simulink model "sysgenCORDICSinCos"  (Simulink 7.7)
settings: Solver=ode45  StartTime=0.0  StopTime=500  RelTol=1e-3
values from neighbouring files (symbols this model uses):
  blue = blue(1:(min_x*min_y))    [makematrix.m]    (also in rgb.mat = [0 0 0 255 255 255 255 255 255 0 0 0 ... (256 elements, 256x)
undefined symbols (not defined in the file or in its folder): Error_Measurement, sysgenCORDIC_lib
libraries: xbsIndex_r4 x95, dspobslib x9, dspstat3 x4, dspswit3 x2, xbsCopyrightNotice_r4 x1, simulink x1
(part 1 of 2)
settings Model: Creator=alexc  LastModifiedBy=douangp
settings DataIOCC: SignalLoggingName=sigsOut
settings OptimizationCC: BlockReduction=off  BooleanDataType=off  InlineInvariantSignals=on  InitFltsAndDblsToZero=on
settings DebuggingCC: SaveWithParameterizedLinksMsg=none  SignalResolutionControl=TryResolveAllWithWarning  SolverPrmCheckMsg=none  MultiTaskDSMMsg=warning  MultiTaskCondExecSysMsg=none  StrictBusMsg=None
settings HardwareCC: TargetUnknown=on
settings RTWCC: IncludeERTFirstTime=on
settings GRTTargetCC: TargetFcnLib=ansi_tfl_tmw.mat

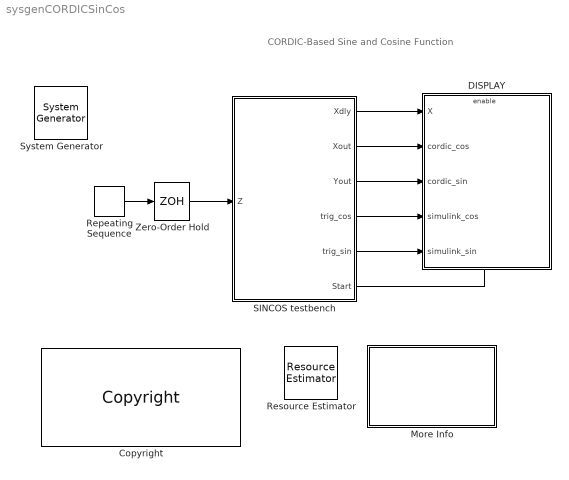
== system sysgenCORDICSinCos ==
  note: CORDIC-Based Sine and Cosine Function
  " System Generator" : xbsIndex_r4/ System Generator  Tag=genX  SystemSampleTime=-1  xilinxfamily=kintex7  part=xc7k325t  speed=-1  package=ffg900  synthesis_tool=XST  clock_wrapper=Clock Enables  directory=./netlist_sysgenCordicSinCos  proj_type=Project Navigator  Synth_file=XST Defaults  Impl_file=ISE Defaults  testbench=off  simulink_period=1  sysclk_period=5  dcm_input_clock_period=100  incr_netlist=off  trim_vbits=Everywhere in SubSystem  dbl_ovrd=According to Block Masks  core_generation=Not Needed - Already Generated  run_coregen=off  deprecated_control=off  eval_field=0  block_type=sysgen
      settings: block_version=9.2.00
  Copyright : xbsCopyrightNotice_r4/Copyright  copyrighttext="Copyright (c) 2011  by  Xilinx, Inc. All rights reserved.<br><br>This file contains proprietary, confidential information of Xilinx, Inc., is distributed under license from Xilinx, Inc., and may be used, copied and/or disclosed only pursuant to the terms of a valid license agreement with Xilinx, Inc. Xilinx hereby grants you a license to use this file solely for design, simulation, implementation and creation of design files limited to Xilinx devices or technologies. Use with non-Xilinx devices or technologies is expressly prohibited and immediately terminates your license unless covered by a separate agreement.<br><br>Xilinx is providing this design, code, or information \"as-is\" solely for use in developing programs and solutions for Xilinx devices, with no obligation on the part of Xilinx to provide support. By providing this design, code, or information as one possible implementation of this feature, application or standard, Xilinx is making no representation that this implementation is free from any claims of infringement. You are responsible for obtaining any rights you may require for your implementation. Xilinx expressly disclaims any warranty whatsoever with respect to the adequacy of the implementation, including but not limited to any warranties or representations that this implementation is free from claims of infringement, implied warranties of merchantability or fitness for a particular purpose.<br><br>Xilinx products are not intended for use in life support appliances, devices, or systems. Use in such applications is expressly prohibited.<br><br>Any modifications that are made to the Source Code are done at the user's sole risk and will be unsupported.<br><br>This copyright and support notice must be retained as part of this text at all times. (c) Copyright 1995-2011 Xilinx, Inc. All rights reserved."  block_type=copyright
      settings: block_version=10.1.00
      settings: infoedit=|
      | Copyright(C) 2008 by  Xilinx, Inc. All rights reserved.<br>
      | <br>
      | This file contains proprietary, confidential information of Xilinx, Inc., is distributed under license
      | from Xilinx, Inc., and may be used, copied and/or disclosed only pursuant to the terms of a valid license
      | agreement with Xilinx, Inc. Xilinx hereby grants you a license to use this file solely for design,
      | simulation, implementation and creation of design files limited to Xilinx devices or technologies. Use
      | with non-Xilinx devices or technologies is expressly prohibited and immediately terminates your license
      | unless covered by a separate agreement.<br>
      | <br>
      | Xilinx is providing this design, code, or information "as-is" solely for use in developing programs and
      | solutions for Xilinx devices, with no obligation on the part of Xilinx to provide support. By providing
      | this design, code, or information as one possible implementation of this feature, application or standard,
      | Xilinx is making no representation that this implementation is free from any claims of infringement. You
      | are responsible for obtaining any rights you may require for your implementation. Xilinx expressly disclaims
      | any warranty whatsoever with respect to the adequacy of the implementation, including but not limited to any
      | warranties or representations that this implementation is free from claims of infringement, implied warranties
      | of merchantability or fitness for a particular purpose.<br>
      | <br>
      | Xilinx products are not intended for use in life support appliances, devices, or systems. Use in such
      | applications is expressly prohibited.<br>
      | <br>
      | Any modifications that are made to the Source Code are done at the user's sole risk and will be unsupported.<br>
      | <br>
      | This copyright and support notice must be retained as part of this text at all times.
      | (c) Copyright 1995-2008 Xilinx, Inc. All rights reserved.
  DISPLAY : Subsystem  TreatAsAtomicUnit=on
  More Info : Subsystem
      mask Display: disp('Double click\n for\n more information.')
  Repeating Sequence : simulink/Sources/Repeating Sequence  SystemSampleTime=-1  rep_seq_t=0:1:201  rep_seq_y=-pi:1/32:pi
  Resource Estimator : xbsIndex_r4/Resource Estimator  Tag=resEstTag  Slices=324  FFs=532  BRAMs=0  LUTs=556  IOBs=48  EBMs=0  TBUFs=0  xl_use_estimator_area=off  est_options=Estimate  xl_estimator_area=[324 532 0 556 48 0 0]  mrp_directory=./sysgenCORDIC_work_test  simulink_period=1  block_type=resource_estimator
      settings: AttributesFormatString=Resource\nEstimator  block_version=9.2.00
  SINCOS testbench : Subsystem  mask{pe_stages=8, pe_nbits=16, pe_binpt=13}
      mask prompts: pe_stages "Number of Processing Stages"; pe_nbits "Number of X, Y, Z Bits"; pe_binpt "X, Y, Z Binary Point Position"
      mask help: CORDIC processor and Simulink conformance testbench. Block parameters allow customization of the CORDIC processor. The number of iteration stages (and resultant output accuracy) and the processor arithmetic precision are controlled by the mask customization.
      mask init:
      | [bg,fg] = xlcmap('XBlock',0);
      | iPos = get_param(gcb,'Position');
      | iWidth=iPos(3)-iPos(1); iHeight=iPos(4)-iPos(2);
      | iCx=iWidth/2;
      | iCy=iHeight/2;
      | [logoX, logoY] = xlogo(iPos);
      | 
      | latency = pe_stages + 5;
      | str = sprintf('-%d',latency);
      mask Help:
      | This design implements a fully parallel CORDIC  (COordinate Rotation DIgital Computer) algorithm in rotational mode that computes
      | the sine and cosine of the input angle z between +/- pi.
      | </p>
      | The CORDIC algorithm is attractive for an FPGA implementation because it consists primarily of shift and add operations.
      | An N-bit adder/subtractor  requiries only N/2 logic slices.  The CORDIC subsystem is masked, and allows customization of bit precision,
      | the number of processing elements (PEs) in the CORDIC engine and the ability to pieline each individual stage.  With eight PEs, the design occupies 503 LUTs (49%),
      | 412 flip-flops (40%), and 272 slices (53%) of a Xilinx xc2v80-5 part. The maximum clock frequency is approximately 230.04 MHz (Device speed data version:
      | PRODUCTION 1.121 2005-11-04, ISE 8.1i software, VHDL synthesized with XST).
      | </p>
      | The CORDIC subsystem is suitable for reuse as a standalone component.
      | </p>
      | <ul>
      | References:
      | <li>J. E. Volder, "The CORDIC Trigonometric Computing Technique", IRE Trans. On Electronic Computers, Vol. EC-8,  1959, pp. 330-334.</li>
      | <li>J. S. Walther, "A Unified Algorithm for Elementary Functions", Spring Joint Computer Conference (1971) pp. 379-385.</li>
      | <li>Yu Hen Hu, "CORDIC-Based VLSI Architectures for Digital Signal Processing", IEEE Signal Processing Magazine, pp. 17-34, July 1992.</li>
      | </ul>
      mask Display:
      | patch([0 iWidth iWidth 0],[0 0 iHeight iHeight] , bg);
      | patch(logoX,logoY , fg);
      | text(iCx-6,iCy,'z');
      | text(iCx,iCy+4,str);
      | port_label('input',1,'z');
      | port_label('output',1,'z_dly');
      | port_label('output',2,'cordic_cos');
      | port_label('output',3,'cordic_sine');
      | port_label('output',4,'simulink_cos');
      | port_label('output',5,'simulink_sin');
      | port_label('output',6,'Start');
      | plot([0 0 iWidth iWidth 0], [0 iHeight iHeight 0 0]);
  Zero-Order Hold : ZeroOrderHold
  wires:
  SINCOS testbench/1(Xdly) -> DISPLAY/1(X)
  SINCOS testbench/4(trig_cos) -> DISPLAY/4(simulink_cos)
  SINCOS testbench/5(trig_sin) -> DISPLAY/5(simulink_sin)
  SINCOS testbench/6(Start) -> DISPLAY/Enable
  Zero-Order Hold/1 -> SINCOS testbench/1(Z)
  Repeating Sequence/1 -> Zero-Order Hold/1
  SINCOS testbench/2(Xout) -> DISPLAY/2(cordic_cos)
  SINCOS testbench/3(Yout) -> DISPLAY/3(cordic_sin)

== system sysgenCORDICSinCos/DISPLAY ==
  note: This subsystem compares the fixed-point CORDIC output with double-precision functions computed in Simulink. The CORDIC OVERLAY scope
      | displays the original input signals and the superposition of the respective output signals.  The Error Measurement subsystems provide additional
      | comparative information.  This enabled subsystem is activated after the number of sample periods equal to the latency of the CORDIC processor.
  X : Inport
  cordic_cos : Inport  Port=2
  cordic_sin : Inport  Port=3
  simulink_cos : Inport  Port=4
  simulink_sin : Inport  Port=5
  Enable : EnablePort
  CORDIC  OVERLAY : Scope  NumInputPorts=3
      settings: TimeRange=500  YMin=-4~-1~-1.5  YMax=4~1.5~1.5
  Mux : Mux  Inputs=2
  Mux1 : Mux  Inputs=2
  cos  Error Measurement : Subsystem  AncestorBlock=sysgenCORDIC_lib/Error_Measurement
      mask Type: Error Measurement
  sin  Error Measurement : Subsystem
      mask Type: Error Measurement
  wires:
  cordic_cos/1 -> Mux/1, cos  Error Measurement/1(In1)
  simulink_cos/1 -> Mux/2, cos  Error Measurement/2(In2)
  X/1 -> CORDIC  OVERLAY/1
  cordic_sin/1 -> Mux1/1, sin  Error Measurement/1(In1)
  simulink_sin/1 -> Mux1/2, sin  Error Measurement/2(In2)
  Mux1/1 -> CORDIC  OVERLAY/3
  Mux/1 -> CORDIC  OVERLAY/2

== system sysgenCORDICSinCos/More Info ==
  note: This design implements a fully parallel CORDIC  (COordinate Rotation DIgital Computer) algorithm in rotational mode that computes
      | the sine and cosine of the input angle z between +/- pi.
      |
      | The CORDIC algorithm is attractive for an FPGA implementation because it consists primarily of shift and add operations.
      | An N-bit adder/subtractor  requiries only N/2 logic slices.  The CORDIC subsystem is masked, and allows customization of bit precision,
      | the number of processing elements (PEs) in the CORDIC engine and the ability to pieline each individual stage.
      |
      | References:
      | J. E. Volder, "The CORDIC Trigonometric Computing Technique", IRE Trans. On Electronic Computers, Vol. EC-8,  1959, pp. 330-334.
      | J. S. Walther, "A Unified Algorithm for Elementary Functions", Spring Joint Computer Conference (1971) pp. 379-385.
      | Yu Hen Hu, "CORDIC-Based VLSI Architectures for Digital Signal Processing", IEEE Signal Processing Magazine, pp. 17-34, July 1992.
  note: CORDIC-Based Sine and Cosine Function

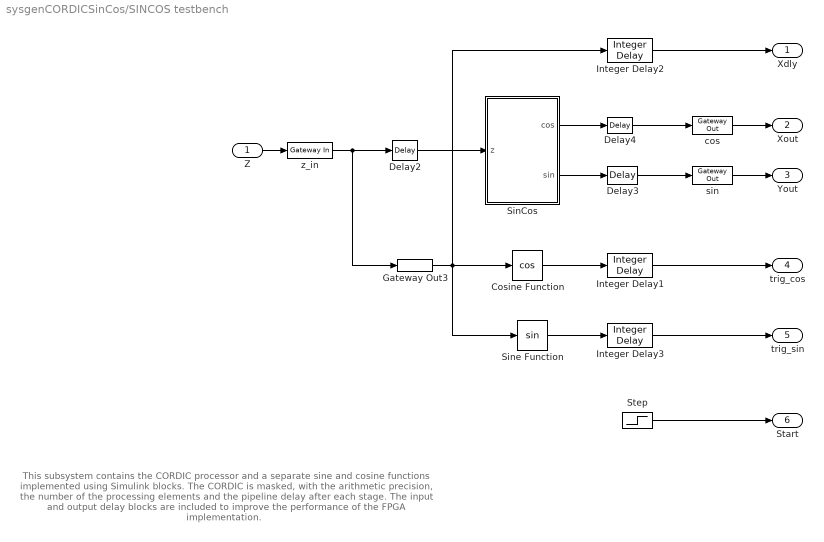
== system sysgenCORDICSinCos/SINCOS testbench ==
  note: This subsystem contains the CORDIC processor and a separate sine and cosine functions implemented using Simulink blocks.
      | The CORDIC is masked, with the arithmetic precision, the number of the processing elements and the pipeline delay after each
      | stage. The input and output delay blocks are included to improve the performance of the FPGA implementation.
  Z : Inport
  Cosine Function : Trigonometry  Operator=cos
  Delay2 : xbsIndex_r4/Delay  rst=off  infoeditControl=Selection of Reset will increase slice count due to use of real FFs and instead of SRLs  en=off  latency=1  dbl_ovrd=off  reg_retiming=off  block_type=delay
      settings: infoedit="Delay line having  configurable length.<P><P>Hardware notes: A delay line is a chain, each link of which is an SRL16 followed by a flip-flop. If register retiming is enabled, the delay line is a chain of flip-flops."  xl_area=[8 16 0 0 0 0 0]  block_version=VER_STRING_GOES_HERE
  Delay3 : xbsIndex_r4/Delay  rst=off  infoeditControl=Selection of Reset will increase slice count due to use of real FFs and instead of SRLs  en=off  latency=1  dbl_ovrd=off  reg_retiming=off  block_type=delay
      settings: infoedit="Delay line having  configurable length.<P><P>Hardware notes: A delay line is a chain, each link of which is an SRL16 followed by a flip-flop. If register retiming is enabled, the delay line is a chain of flip-flops."  xl_area=[8 16 0 0 0 0 0]  block_version=VER_STRING_GOES_HERE
  Delay4 : xbsIndex_r4/Delay  rst=off  infoeditControl=Selection of Reset will increase slice count due to use of real FFs and instead of SRLs  en=off  latency=1  dbl_ovrd=off  reg_retiming=off  block_type=delay
      settings: infoedit="Delay line having  configurable length.<P><P>Hardware notes: A delay line is a chain, each link of which is an SRL16 followed by a flip-flop. If register retiming is enabled, the delay line is a chain of flip-flops."  xl_area=[8 16 0 0 0 0 0]  block_version=VER_STRING_GOES_HERE
  Gateway Out3 : xbsIndex_r4/Gateway Out  hdl_port=off  timing_constraint=None  locs_specified=off  LOCs={}  block_type=gatewayout
      settings: infoedit="Gateway out block.  Converts Xilinx fixed point inputs into ouputs of type Simulink integer, double, or fixed point.<P><P>Hardware notes:  In hardware these blocks become top level output ports or are discarded, depending on how they are configured."  xl_area=[0 0 0 0 0 0 0]  block_version=VER_STRING_GOES_HERE
  Integer Delay1 : dspobslib/Integer Delay  delay=latency  ic=0  reset_popup=None
  Integer Delay2 : dspobslib/Integer Delay  delay=latency  ic=0  reset_popup=None
  Integer Delay3 : dspobslib/Integer Delay  delay=latency  ic=0  reset_popup=None
  SinCos : Subsystem  mask{pe_stages=pe_stages, pe_nbits=pe_nbits, pe_binpt=pe_binpt, sg_icon_stat=80,126,1,3,white,blue,0,,right}
      mask prompts: pe_stages "Stages"; pe_nbits "Number of bits"; pe_binpt "Binary point position"; sg_icon_stat "Mask Parameter 4:"
      mask init:
      | xBlock(struct('source', str2func('cordic_sincos_script'), 'toplevel', gcb, 'depend', {{'cordic_sincos_script'}}), {pe_stages, pe_nbits, pe_binpt});
      mask Display:
      | fprintf('','COMMENT: begin icon graphics');
      | patch([0 70 70 0 ],[0 0 104 104 ],[0.77 0.82 0.91]);
      | patch([17 5 21 5 17 35 40 45 65 49 34 23 39 23 34 49 65 45 40 35 17 ],[25 37 53 69 81 81 76 81 81 65 80 69 53 37 26 41 25 25 30 25 25 ],[0.98 0.96 0.92]);
      | plot([0 70 70 0 0 ],[0 0 104 104 0 ]);
      | fprintf('','COMMENT: end icon graphics');
      | fprintf('','COMMENT: begin icon text');
      | color('black');port_label('input',1,'z');
      | color('black');port_label('output',1,'cos');
      | color('black');port_label('output',2,'sin');
      | fprintf('','COMMENT: end icon text');
  Sine Function : Trigonometry
  Step : Step  Time=latency  SampleTime=1
  cos : xbsIndex_r4/Gateway Out  hdl_port=on  timing_constraint=None  locs_specified=off  LOCs={}  block_type=gatewayout
      settings: infoedit="Gateway out block.  Converts Xilinx fixed point inputs into ouputs of type Simulink integer, double, or fixed point.<P><P>Hardware notes:  In hardware these blocks become top level output ports or are discarded, depending on how they are configured."  xl_area=[0 0 0 0 16 0 0]  block_version=VER_STRING_GOES_HERE
  sin : xbsIndex_r4/Gateway Out  hdl_port=on  timing_constraint=None  locs_specified=off  LOCs={}  block_type=gatewayout
      settings: infoedit="Gateway out block.  Converts Xilinx fixed point inputs into ouputs of type Simulink integer, double, or fixed point.<P><P>Hardware notes:  In hardware these blocks become top level output ports or are discarded, depending on how they are configured."  xl_area=[0 0 0 0 16 0 0]  block_version=VER_STRING_GOES_HERE
  z_in : xbsIndex_r4/Gateway In  gui_display_data_type=Fixed-point  arith_type="Signed  (2's comp)"  n_bits=pe_nbits  bin_pt=pe_binpt  preci_type=Single  exp_width=8  frac_width=24  quantization="Round  (unbiased: +/- Inf)"  overflow=Saturate  period=1  dbl_ovrd=off  timing_constraint=None  locs_specified=off  LOCs={}  hdl_port=on  block_type=gatewayin
      settings: infoedit="Gateway in block.  Converts inputs of type Simulink integer, double and fixed point to  Xilinx fixed point type.<P><P>Hardware notes:  In hardware these blocks become top level input ports."  xl_area=[0 0 0 0 16 0 0]  block_version=VER_STRING_GOES_HERE
  Xdly : Outport
  Xout : Outport  Port=2
  Yout : Outport  Port=3
  trig_cos : Outport  Port=4
  trig_sin : Outport  Port=5
  Start : Outport  Port=6
  wires:
  Gateway Out3/1 -> Sine Function/1, Cosine Function/1, Integer Delay2/1
  Step/1 -> Start/1
  Integer Delay3/1 -> trig_sin/1
  Integer Delay1/1 -> trig_cos/1
  sin/1 -> Yout/1
  cos/1 -> Xout/1
  Sine Function/1 -> Integer Delay3/1
  Delay4/1 -> cos/1
  Z/1 -> z_in/1
  Integer Delay2/1 -> Xdly/1
  Delay3/1 -> sin/1
  Delay2/1 -> SinCos/1(z)
  Cosine Function/1 -> Integer Delay1/1
  z_in/1 -> Gateway Out3/1, Delay2/1
  SinCos/1(cos) -> Delay4/1
  SinCos/2(sin) -> Delay3/1

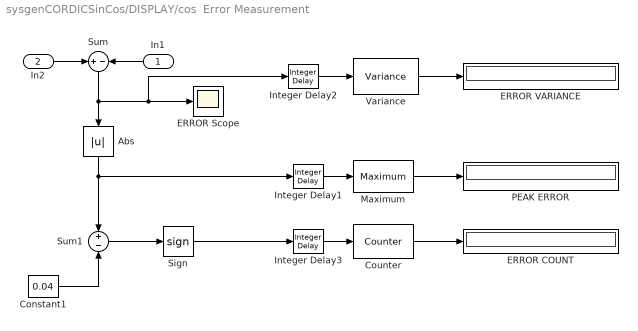
== system sysgenCORDICSinCos/DISPLAY/cos  Error Measurement ==
  In1 : Inport
  In2 : Inport  Port=2
  Abs : Abs  SaturateOnIntegerOverflow=on
  Constant1 : Constant  Value=0.04
  Counter : dspswit3/Counter  Direction=Up  CountEvent=Rising edge  CounterSize=User defined  MaxCount=200000000  InitialCount=0  Output=Count  HitValue=32  ResetInput=off  SamplesPerFrame=1  Ts=1  CntDtype=double  HitDtype=Logical
  ERROR Scope : Scope
      settings: TimeRange=10000  YMin=-0.0006  YMax=0.0005  SaveName=ScopeData2
  ERROR COUNT : Display
      settings: Format=long_e
  ERROR VARIANCE : Display
      settings: Format=long_e
  Integer Delay1 : dspobslib/Integer Delay  delay=1  ic=0  reset_popup=None
  Integer Delay2 : dspobslib/Integer Delay  delay=1  ic=0  reset_popup=None
  Integer Delay3 : dspobslib/Integer Delay  delay=1  ic=0  reset_popup=None
  Maximum : dspstat3/Maximum  fcn=Running  reset=None  InputProcessing=Inherited (this choice will be removed - see release notes)  indexBase=One  operateOver=Each column  Dimension=1  colComp=on  operation=maximum  roiEnable=off  roiType=Rectangles  roiPortion=Entire ROI  roiOutput=Individual statistics for each ROI  roiFlag=off  accumDataTypeStr=Inherit: Same as product output  accumLastDataTypeStr=Inherit: Same as product output  roundingMode=Floor  overflowMode=off
  PEAK ERROR : Display
      settings: Format=long_e
  Sign : Signum
  Sum : Sum  Inputs=+-  SaturateOnIntegerOverflow=on  InputSameDT=on  OutDataTypeStr=Inherit: Same as first input
  Sum1 : Sum  Inputs=+-  SaturateOnIntegerOverflow=on  InputSameDT=on  OutDataTypeStr=Inherit: Same as first input
  Variance : dspstat3/Variance  run=on  reset_popup=None  InputProcessing=Inherited (this choice will be removed - see release notes)  directionMode=Each column  dimension=1  treatSBRowAsCol=on  roiEnable=off  roiType=Rectangles  roiPortion=Entire ROI  roiOutput=Individual statistics for each ROI  roiFlag=off  roundingMode=Floor  overflowMode=off
  wires:
  Sum/1 -> Abs/1, ERROR Scope/1, Integer Delay2/1
  Constant1/1 -> Sum1/2
  Abs/1 -> Sum1/1, Integer Delay1/1
  Sum1/1 -> Sign/1
  Sign/1 -> Integer Delay3/1
  Counter/1 -> ERROR COUNT/1
  Variance/1 -> ERROR VARIANCE/1
  Maximum/1 -> PEAK ERROR/1
  Integer Delay3/1 -> Counter/1
  Integer Delay1/1 -> Maximum/1
  Integer Delay2/1 -> Variance/1
  In1/1 -> Sum/2
  In2/1 -> Sum/1

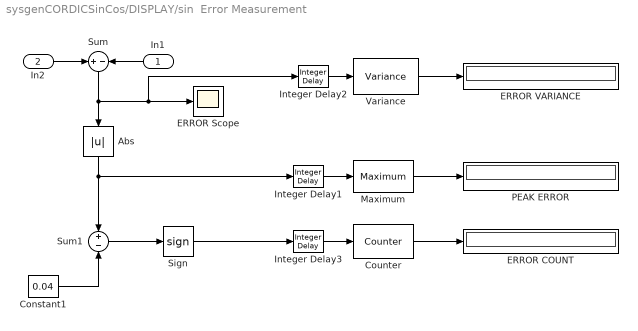
== system sysgenCORDICSinCos/DISPLAY/sin  Error Measurement ==
  In1 : Inport
  In2 : Inport  Port=2
  Abs : Abs  SaturateOnIntegerOverflow=on
  Constant1 : Constant  Value=0.04
  Counter : dspswit3/Counter  Direction=Up  CountEvent=Rising edge  CounterSize=User defined  MaxCount=200000000  InitialCount=0  Output=Count  HitValue=32  ResetInput=off  SamplesPerFrame=1  Ts=1  CntDtype=double  HitDtype=Logical
  ERROR Scope : Scope
      settings: TimeRange=10000  YMin=-0.0006  YMax=0.0005  SaveName=ScopeData2
  ERROR COUNT : Display
      settings: Format=long_e
  ERROR VARIANCE : Display
      settings: Format=long_e
  Integer Delay1 : dspobslib/Integer Delay  delay=1  ic=0  reset_popup=None
  Integer Delay2 : dspobslib/Integer Delay  delay=1  ic=0  reset_popup=None
  Integer Delay3 : dspobslib/Integer Delay  delay=1  ic=0  reset_popup=None
  Maximum : dspstat3/Maximum  fcn=Running  reset=None  InputProcessing=Inherited (this choice will be removed - see release notes)  indexBase=One  operateOver=Each column  Dimension=1  colComp=on  operation=maximum  roiEnable=off  roiType=Rectangles  roiPortion=Entire ROI  roiOutput=Individual statistics for each ROI  roiFlag=off  accumDataTypeStr=Inherit: Same as product output  accumLastDataTypeStr=Inherit: Same as product output  roundingMode=Floor  overflowMode=off
  PEAK ERROR : Display
      settings: Format=long_e
  Sign : Signum
  Sum : Sum  Inputs=+-  SaturateOnIntegerOverflow=on  InputSameDT=on  OutDataTypeStr=Inherit: Same as first input
  Sum1 : Sum  Inputs=+-  SaturateOnIntegerOverflow=on  InputSameDT=on  OutDataTypeStr=Inherit: Same as first input
  Variance : dspstat3/Variance  run=on  reset_popup=None  InputProcessing=Inherited (this choice will be removed - see release notes)  directionMode=Each column  dimension=1  treatSBRowAsCol=on  roiEnable=off  roiType=Rectangles  roiPortion=Entire ROI  roiOutput=Individual statistics for each ROI  roiFlag=off  roundingMode=Floor  overflowMode=off
  wires:
  Sum/1 -> Abs/1, ERROR Scope/1, Integer Delay2/1
  Constant1/1 -> Sum1/2
  Abs/1 -> Sum1/1, Integer Delay1/1
  Sum1/1 -> Sign/1
  Sign/1 -> Integer Delay3/1
  Counter/1 -> ERROR COUNT/1
  Variance/1 -> ERROR VARIANCE/1
  Maximum/1 -> PEAK ERROR/1
  Integer Delay3/1 -> Counter/1
  Integer Delay1/1 -> Maximum/1
  Integer Delay2/1 -> Variance/1
  In1/1 -> Sum/2
  In2/1 -> Sum/1

== system sysgenCORDICSinCos/SINCOS testbench/SinCos ==
  z : Inport
  Constant2 : xbsIndex_r4/Constant  const=0.607253030192621  gui_display_data_type=Fixed-point  arith_type=Signed (2's comp)  n_bits=16  bin_pt=13  preci_type=Single  exp_width=8  frac_width=24  explicit_period=off  period=1  equ=P=C  opselect=C  inp2=PCIN>>17  opr=+  inp1=P  carry=CIN  dbl_ovrd=off  block_type=constant
  Constant3 : xbsIndex_r4/Constant  const=0  gui_display_data_type=Fixed-point  arith_type=Signed (2's comp)  n_bits=16  bin_pt=13  preci_type=Single  exp_width=8  frac_width=24  explicit_period=off  period=1  equ=P=C  opselect=C  inp2=PCIN>>17  opr=+  inp1=P  carry=CIN  dbl_ovrd=off  block_type=constant
  Delay1 : xbsIndex_r4/Delay  rst=off  infoeditControl=Selection of Reset will increase slice count due to use of real FFs and instead of SRLs  en=off  latency=9  dbl_ovrd=off  reg_retiming=off  block_type=delay
  Delay2 : xbsIndex_r4/Delay  rst=off  infoeditControl=Selection of Reset will increase slice count due to use of real FFs and instead of SRLs  en=off  latency=10  dbl_ovrd=off  reg_retiming=off  block_type=delay
  fine_angle_pe : Subsystem
  quandrant_correct : Subsystem
  quandrant_map : Subsystem
  cos : Outport
  sin : Outport  Port=2
  wires:
  quandrant_correct/2(sine) -> sin/1
  quandrant_correct/1(cosine) -> cos/1
  Delay2/1 -> quandrant_correct/4(sgn_z)
  Delay1/1 -> quandrant_correct/3(angle_map)
  fine_angle_pe/2(out1) -> quandrant_correct/2(s)
  fine_angle_pe/1(out0) -> quandrant_correct/1(c)
  quandrant_map/3(sgn_z) -> Delay2/1
  quandrant_map/2(angle_map) -> Delay1/1
  quandrant_map/1(zo) -> fine_angle_pe/3(in2)
  Constant3/1 -> fine_angle_pe/2(in1)
  Constant2/1 -> fine_angle_pe/1(in0)
  z/1 -> quandrant_map/1(z)

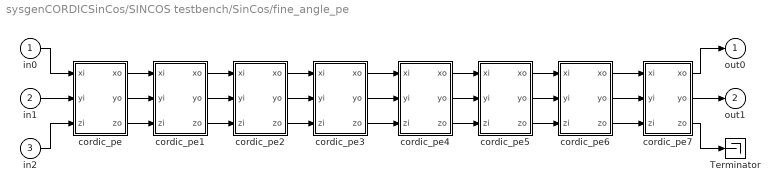
== system sysgenCORDICSinCos/SINCOS testbench/SinCos/fine_angle_pe ==
  in0 : Inport
  in1 : Inport  Port=2
  in2 : Inport  Port=3
  Terminator : Terminator
  cordic_pe : Subsystem
  cordic_pe1 : Subsystem
  cordic_pe2 : Subsystem
  cordic_pe3 : Subsystem
  cordic_pe4 : Subsystem
  cordic_pe5 : Subsystem
  cordic_pe6 : Subsystem
  cordic_pe7 : Subsystem
  out0 : Outport
  out1 : Outport  Port=2
  wires:
  cordic_pe7/3(zo) -> Terminator/1
  cordic_pe7/2(yo) -> out1/1
  cordic_pe7/1(xo) -> out0/1
  cordic_pe6/3(zo) -> cordic_pe7/3(zi)
  cordic_pe6/2(yo) -> cordic_pe7/2(yi)
  cordic_pe6/1(xo) -> cordic_pe7/1(xi)
  cordic_pe5/3(zo) -> cordic_pe6/3(zi)
  cordic_pe5/2(yo) -> cordic_pe6/2(yi)
  cordic_pe5/1(xo) -> cordic_pe6/1(xi)
  cordic_pe4/3(zo) -> cordic_pe5/3(zi)
  cordic_pe4/2(yo) -> cordic_pe5/2(yi)
  cordic_pe4/1(xo) -> cordic_pe5/1(xi)
  cordic_pe3/3(zo) -> cordic_pe4/3(zi)
  cordic_pe3/2(yo) -> cordic_pe4/2(yi)
  cordic_pe3/1(xo) -> cordic_pe4/1(xi)
  cordic_pe2/3(zo) -> cordic_pe3/3(zi)
  cordic_pe2/2(yo) -> cordic_pe3/2(yi)
  cordic_pe2/1(xo) -> cordic_pe3/1(xi)
  cordic_pe1/3(zo) -> cordic_pe2/3(zi)
  cordic_pe1/2(yo) -> cordic_pe2/2(yi)
  cordic_pe1/1(xo) -> cordic_pe2/1(xi)
  cordic_pe/3(zo) -> cordic_pe1/3(zi)
  cordic_pe/2(yo) -> cordic_pe1/2(yi)
  cordic_pe/1(xo) -> cordic_pe1/1(xi)
  in2/1 -> cordic_pe/3(zi)
  in1/1 -> cordic_pe/2(yi)
  in0/1 -> cordic_pe/1(xi)

== system sysgenCORDICSinCos/SINCOS testbench/SinCos/quandrant_correct ==
  c : Inport
  s : Inport  Port=2
  angle_map : Inport  Port=3
  sgn_z : Inport  Port=4
  Mux1 : xbsIndex_r4/Mux  inputs=2  en=off  latency=0  precision=Full  arith_type=Unsigned  n_bits=16  bin_pt=14  quantization=Truncate  overflow=Wrap  dbl_ovrd=off  block_type=mux
  Mux2 : xbsIndex_r4/Mux  inputs=2  en=off  latency=0  precision=Full  arith_type=Unsigned  n_bits=16  bin_pt=14  quantization=Truncate  overflow=Wrap  dbl_ovrd=off  block_type=mux
  Mux3 : xbsIndex_r4/Mux  inputs=2  en=off  latency=1  precision=Full  arith_type=Unsigned  n_bits=16  bin_pt=14  quantization=Truncate  overflow=Wrap  dbl_ovrd=off  block_type=mux
  Mux4 : xbsIndex_r4/Mux  inputs=2  en=off  latency=1  precision=Full  arith_type=Unsigned  n_bits=16  bin_pt=14  quantization=Truncate  overflow=Wrap  dbl_ovrd=off  block_type=mux
  Negate : xbsIndex_r4/Negate  precision=User Defined  arith_type="Signed  (2's comp)"  n_bits=16  bin_pt=13  quantization=Truncate  overflow=Wrap  en=off  latency=0  dbl_ovrd=off  block_type=negate
  Negate1 : xbsIndex_r4/Negate  precision=User Defined  arith_type="Signed  (2's comp)"  n_bits=16  bin_pt=13  quantization=Truncate  overflow=Wrap  en=off  latency=0  dbl_ovrd=off  block_type=negate
  cosine : Outport
  sine : Outport  Port=2
  wires:
  s/1 -> Mux4/2, Mux1/3, Negate/1
  sgn_z/1 -> Mux2/1, Mux1/1
  c/1 -> Mux3/2, Mux2/2, Negate1/1
  angle_map/1 -> Mux4/1, Mux3/1
  Mux4/1 -> sine/1
  Mux2/1 -> Mux4/3
  Mux3/1 -> cosine/1
  Mux1/1 -> Mux3/3
  Negate1/1 -> Mux2/3
  Negate/1 -> Mux1/2

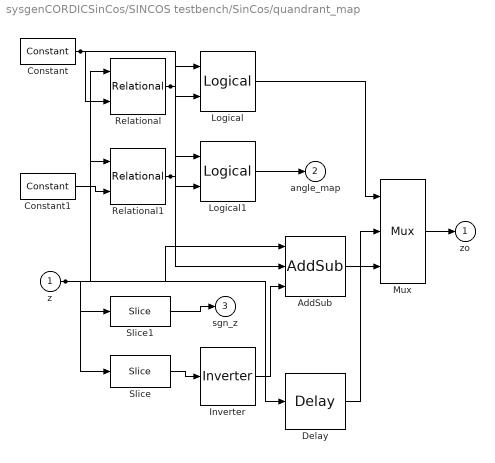
== system sysgenCORDICSinCos/SINCOS testbench/SinCos/quandrant_map ==
  z : Inport
  AddSub : xbsIndex_r4/AddSub  mode=Addition or Subtraction  use_carryin=off  use_carryout=off  en=off  latency=1  precision=User Defined  arith_type="Signed  (2's comp)"  n_bits=16  bin_pt=13  quantization=Truncate  overflow=Wrap  dbl_ovrd=off  use_behavioral_HDL=off  hw_selection=Fabric  pipelined=off  block_type=addsub
  Constant : xbsIndex_r4/Constant  const=1.5707963267949  gui_display_data_type=Fixed-point  arith_type=Signed (2's comp)  n_bits=16  bin_pt=13  preci_type=Single  exp_width=8  frac_width=24  explicit_period=off  period=1  equ=P=C  opselect=C  inp2=PCIN>>17  opr=+  inp1=P  carry=CIN  dbl_ovrd=off  block_type=constant
  Constant1 : xbsIndex_r4/Constant  const=-1.5707963267949  gui_display_data_type=Fixed-point  arith_type=Signed (2's comp)  n_bits=16  bin_pt=13  preci_type=Single  exp_width=8  frac_width=24  explicit_period=off  period=1  equ=P=C  opselect=C  inp2=PCIN>>17  opr=+  inp1=P  carry=CIN  dbl_ovrd=off  block_type=constant
  Delay : xbsIndex_r4/Delay  rst=off  infoeditControl=Selection of Reset will increase slice count due to use of real FFs and instead of SRLs  en=off  latency=1  dbl_ovrd=off  reg_retiming=off  block_type=delay
  Inverter : xbsIndex_r4/Inverter  en=off  latency=0  dbl_ovrd=off  block_type=inv
  Logical : xbsIndex_r4/Logical  logical_function=OR  inputs=2  en=off  latency=0  precision=Full  arith_type=Unsigned  n_bits=16  bin_pt=0  align_bp=on  dbl_ovrd=off  block_type=logical
  Logical1 : xbsIndex_r4/Logical  logical_function=OR  inputs=2  en=off  latency=0  precision=Full  arith_type=Unsigned  n_bits=16  bin_pt=0  align_bp=on  dbl_ovrd=off  block_type=logical
  Mux : xbsIndex_r4/Mux  inputs=2  en=off  latency=1  precision=Full  arith_type=Unsigned  n_bits=16  bin_pt=14  quantization=Truncate  overflow=Wrap  dbl_ovrd=off  block_type=mux
  Relational : xbsIndex_r4/Relational  mode=a>b  en=off  latency=1  dbl_ovrd=off  block_type=relational
  Relational1 : xbsIndex_r4/Relational  mode=a<b  en=off  latency=1  dbl_ovrd=off  block_type=relational
  Slice : xbsIndex_r4/Slice  nbits=1  boolean_output=on  mode=Upper Bit Location + Width  bit1=0  base1=MSB of Input  bit0=0  base0=LSB of Input  dbl_ovrd=off  block_type=slice
  Slice1 : xbsIndex_r4/Slice  nbits=1  boolean_output=on  mode=Upper Bit Location + Width  bit1=0  base1=MSB of Input  bit0=0  base0=LSB of Input  dbl_ovrd=off  block_type=slice
  zo : Outport
  angle_map : Outport  Port=2
  sgn_z : Outport  Port=3
  wires:
  z/1 -> Slice1/1, AddSub/1, Slice/1, Delay/1, Relational1/1, Relational/1
  Constant/1 -> AddSub/2, Relational/2
  Relational/1 -> Logical1/1, Logical/1
  Relational1/1 -> Logical1/2, Logical/2
  Slice1/1 -> sgn_z/1
  Logical1/1 -> angle_map/1
  Mux/1 -> zo/1
  AddSub/1 -> Mux/3
  Delay/1 -> Mux/2
  Logical/1 -> Mux/1
  Inverter/1 -> AddSub/3
  Slice/1 -> Inverter/1
  Constant1/1 -> Relational1/2

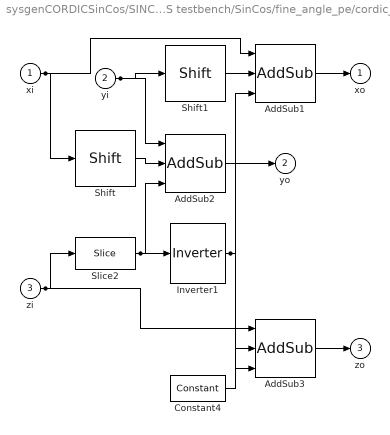
== system sysgenCORDICSinCos/SINCOS testbench/SinCos/fine_angle_pe/cordic_pe ==
  xi : Inport
  yi : Inport  Port=2
  zi : Inport  Port=3
  AddSub1 : xbsIndex_r4/AddSub  mode=Addition or Subtraction  use_carryin=off  use_carryout=off  en=off  latency=1  precision=User Defined  arith_type="Signed  (2's comp)"  n_bits=16  bin_pt=13  quantization=Truncate  overflow=Wrap  dbl_ovrd=off  use_behavioral_HDL=off  hw_selection=Fabric  pipelined=off  block_type=addsub
  AddSub2 : xbsIndex_r4/AddSub  mode=Addition or Subtraction  use_carryin=off  use_carryout=off  en=off  latency=1  precision=User Defined  arith_type="Signed  (2's comp)"  n_bits=16  bin_pt=13  quantization=Truncate  overflow=Wrap  dbl_ovrd=off  use_behavioral_HDL=off  hw_selection=Fabric  pipelined=off  block_type=addsub
  AddSub3 : xbsIndex_r4/AddSub  mode=Addition or Subtraction  use_carryin=off  use_carryout=off  en=off  latency=1  precision=User Defined  arith_type="Signed  (2's comp)"  n_bits=16  bin_pt=13  quantization=Truncate  overflow=Wrap  dbl_ovrd=off  use_behavioral_HDL=off  hw_selection=Fabric  pipelined=off  block_type=addsub
  Constant4 : xbsIndex_r4/Constant  const=0.785398163397448  gui_display_data_type=Fixed-point  arith_type=Signed (2's comp)  n_bits=16  bin_pt=13  preci_type=Single  exp_width=8  frac_width=24  explicit_period=off  period=1  equ=P=C  opselect=C  inp2=PCIN>>17  opr=+  inp1=P  carry=CIN  dbl_ovrd=off  block_type=constant
  Inverter1 : xbsIndex_r4/Inverter  en=off  latency=0  dbl_ovrd=off  block_type=inv
  Shift : xbsIndex_r4/Shift  shift_dir=Right  shift_bits=0  en=off  latency=0  precision=User Defined  arith_type="Signed  (2's comp)"  n_bits=16  bin_pt=13  quantization=Truncate  overflow=Wrap  dbl_ovrd=off  block_type=shift
  Shift1 : xbsIndex_r4/Shift  shift_dir=Right  shift_bits=0  en=off  latency=0  precision=User Defined  arith_type="Signed  (2's comp)"  n_bits=16  bin_pt=13  quantization=Truncate  overflow=Wrap  dbl_ovrd=off  block_type=shift
  Slice2 : xbsIndex_r4/Slice  nbits=1  boolean_output=on  mode=Upper Bit Location + Width  bit1=0  base1=MSB of Input  bit0=0  base0=LSB of Input  dbl_ovrd=off  block_type=slice
  xo : Outport
  yo : Outport  Port=2
  zo : Outport  Port=3
  wires:
  xi/1 -> AddSub1/1, Shift/1
  yi/1 -> AddSub2/1, Shift1/1
  zi/1 -> AddSub3/1, Slice2/1
  Slice2/1 -> AddSub2/3, Inverter1/1
  Inverter1/1 -> AddSub3/3, AddSub1/3
  AddSub3/1 -> zo/1
  Constant4/1 -> AddSub3/2
  AddSub2/1 -> yo/1
  Shift/1 -> AddSub2/2
  AddSub1/1 -> xo/1
  Shift1/1 -> AddSub1/2

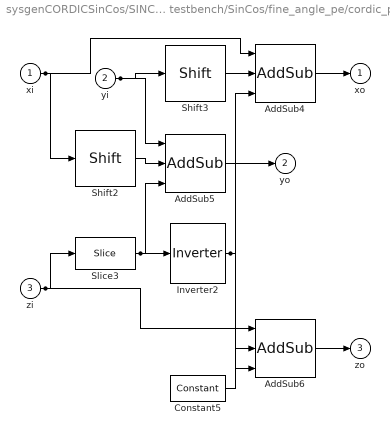
== system sysgenCORDICSinCos/SINCOS testbench/SinCos/fine_angle_pe/cordic_pe1 ==
  xi : Inport
  yi : Inport  Port=2
  zi : Inport  Port=3
  AddSub4 : xbsIndex_r4/AddSub  mode=Addition or Subtraction  use_carryin=off  use_carryout=off  en=off  latency=1  precision=User Defined  arith_type="Signed  (2's comp)"  n_bits=16  bin_pt=13  quantization=Truncate  overflow=Wrap  dbl_ovrd=off  use_behavioral_HDL=off  hw_selection=Fabric  pipelined=off  block_type=addsub
  AddSub5 : xbsIndex_r4/AddSub  mode=Addition or Subtraction  use_carryin=off  use_carryout=off  en=off  latency=1  precision=User Defined  arith_type="Signed  (2's comp)"  n_bits=16  bin_pt=13  quantization=Truncate  overflow=Wrap  dbl_ovrd=off  use_behavioral_HDL=off  hw_selection=Fabric  pipelined=off  block_type=addsub
  AddSub6 : xbsIndex_r4/AddSub  mode=Addition or Subtraction  use_carryin=off  use_carryout=off  en=off  latency=1  precision=User Defined  arith_type="Signed  (2's comp)"  n_bits=16  bin_pt=13  quantization=Truncate  overflow=Wrap  dbl_ovrd=off  use_behavioral_HDL=off  hw_selection=Fabric  pipelined=off  block_type=addsub
  Constant5 : xbsIndex_r4/Constant  const=0.463647609000806  gui_display_data_type=Fixed-point  arith_type=Signed (2's comp)  n_bits=16  bin_pt=13  preci_type=Single  exp_width=8  frac_width=24  explicit_period=off  period=1  equ=P=C  opselect=C  inp2=PCIN>>17  opr=+  inp1=P  carry=CIN  dbl_ovrd=off  block_type=constant
  Inverter2 : xbsIndex_r4/Inverter  en=off  latency=0  dbl_ovrd=off  block_type=inv
  Shift2 : xbsIndex_r4/Shift  shift_dir=Right  shift_bits=1  en=off  latency=0  precision=User Defined  arith_type="Signed  (2's comp)"  n_bits=16  bin_pt=13  quantization=Truncate  overflow=Wrap  dbl_ovrd=off  block_type=shift
  Shift3 : xbsIndex_r4/Shift  shift_dir=Right  shift_bits=1  en=off  latency=0  precision=User Defined  arith_type="Signed  (2's comp)"  n_bits=16  bin_pt=13  quantization=Truncate  overflow=Wrap  dbl_ovrd=off  block_type=shift
  Slice3 : xbsIndex_r4/Slice  nbits=1  boolean_output=on  mode=Upper Bit Location + Width  bit1=0  base1=MSB of Input  bit0=0  base0=LSB of Input  dbl_ovrd=off  block_type=slice
  xo : Outport
  yo : Outport  Port=2
  zo : Outport  Port=3
  wires:
  xi/1 -> AddSub4/1, Shift2/1
  yi/1 -> AddSub5/1, Shift3/1
  zi/1 -> AddSub6/1, Slice3/1
  Slice3/1 -> AddSub5/3, Inverter2/1
  Inverter2/1 -> AddSub6/3, AddSub4/3
  AddSub6/1 -> zo/1
  Constant5/1 -> AddSub6/2
  AddSub5/1 -> yo/1
  Shift2/1 -> AddSub5/2
  AddSub4/1 -> xo/1
  Shift3/1 -> AddSub4/2

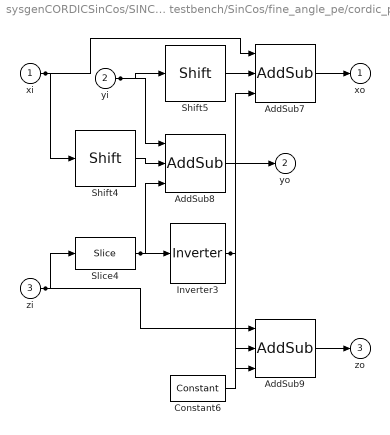
== system sysgenCORDICSinCos/SINCOS testbench/SinCos/fine_angle_pe/cordic_pe2 ==
  xi : Inport
  yi : Inport  Port=2
  zi : Inport  Port=3
  AddSub7 : xbsIndex_r4/AddSub  mode=Addition or Subtraction  use_carryin=off  use_carryout=off  en=off  latency=1  precision=User Defined  arith_type="Signed  (2's comp)"  n_bits=16  bin_pt=13  quantization=Truncate  overflow=Wrap  dbl_ovrd=off  use_behavioral_HDL=off  hw_selection=Fabric  pipelined=off  block_type=addsub
  AddSub8 : xbsIndex_r4/AddSub  mode=Addition or Subtraction  use_carryin=off  use_carryout=off  en=off  latency=1  precision=User Defined  arith_type="Signed  (2's comp)"  n_bits=16  bin_pt=13  quantization=Truncate  overflow=Wrap  dbl_ovrd=off  use_behavioral_HDL=off  hw_selection=Fabric  pipelined=off  block_type=addsub
  AddSub9 : xbsIndex_r4/AddSub  mode=Addition or Subtraction  use_carryin=off  use_carryout=off  en=off  latency=1  precision=User Defined  arith_type="Signed  (2's comp)"  n_bits=16  bin_pt=13  quantization=Truncate  overflow=Wrap  dbl_ovrd=off  use_behavioral_HDL=off  hw_selection=Fabric  pipelined=off  block_type=addsub
  Constant6 : xbsIndex_r4/Constant  const=0.244978663126864  gui_display_data_type=Fixed-point  arith_type=Signed (2's comp)  n_bits=16  bin_pt=13  preci_type=Single  exp_width=8  frac_width=24  explicit_period=off  period=1  equ=P=C  opselect=C  inp2=PCIN>>17  opr=+  inp1=P  carry=CIN  dbl_ovrd=off  block_type=constant
  Inverter3 : xbsIndex_r4/Inverter  en=off  latency=0  dbl_ovrd=off  block_type=inv
  Shift4 : xbsIndex_r4/Shift  shift_dir=Right  shift_bits=2  en=off  latency=0  precision=User Defined  arith_type="Signed  (2's comp)"  n_bits=16  bin_pt=13  quantization=Truncate  overflow=Wrap  dbl_ovrd=off  block_type=shift
  Shift5 : xbsIndex_r4/Shift  shift_dir=Right  shift_bits=2  en=off  latency=0  precision=User Defined  arith_type="Signed  (2's comp)"  n_bits=16  bin_pt=13  quantization=Truncate  overflow=Wrap  dbl_ovrd=off  block_type=shift
  Slice4 : xbsIndex_r4/Slice  nbits=1  boolean_output=on  mode=Upper Bit Location + Width  bit1=0  base1=MSB of Input  bit0=0  base0=LSB of Input  dbl_ovrd=off  block_type=slice
  xo : Outport
  yo : Outport  Port=2
  zo : Outport  Port=3
  wires:
  xi/1 -> AddSub7/1, Shift4/1
  yi/1 -> AddSub8/1, Shift5/1
  zi/1 -> AddSub9/1, Slice4/1
  Slice4/1 -> AddSub8/3, Inverter3/1
  Inverter3/1 -> AddSub9/3, AddSub7/3
  AddSub9/1 -> zo/1
  Constant6/1 -> AddSub9/2
  AddSub8/1 -> yo/1
  Shift4/1 -> AddSub8/2
  AddSub7/1 -> xo/1
  Shift5/1 -> AddSub7/2

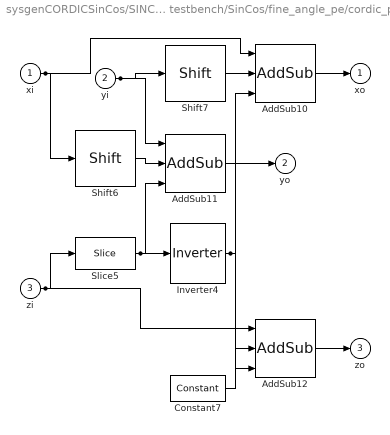
== system sysgenCORDICSinCos/SINCOS testbench/SinCos/fine_angle_pe/cordic_pe3 ==
  xi : Inport
  yi : Inport  Port=2
  zi : Inport  Port=3
  AddSub10 : xbsIndex_r4/AddSub  mode=Addition or Subtraction  use_carryin=off  use_carryout=off  en=off  latency=1  precision=User Defined  arith_type="Signed  (2's comp)"  n_bits=16  bin_pt=13  quantization=Truncate  overflow=Wrap  dbl_ovrd=off  use_behavioral_HDL=off  hw_selection=Fabric  pipelined=off  block_type=addsub
  AddSub11 : xbsIndex_r4/AddSub  mode=Addition or Subtraction  use_carryin=off  use_carryout=off  en=off  latency=1  precision=User Defined  arith_type="Signed  (2's comp)"  n_bits=16  bin_pt=13  quantization=Truncate  overflow=Wrap  dbl_ovrd=off  use_behavioral_HDL=off  hw_selection=Fabric  pipelined=off  block_type=addsub
  AddSub12 : xbsIndex_r4/AddSub  mode=Addition or Subtraction  use_carryin=off  use_carryout=off  en=off  latency=1  precision=User Defined  arith_type="Signed  (2's comp)"  n_bits=16  bin_pt=13  quantization=Truncate  overflow=Wrap  dbl_ovrd=off  use_behavioral_HDL=off  hw_selection=Fabric  pipelined=off  block_type=addsub
  Constant7 : xbsIndex_r4/Constant  const=0.124354994546761  gui_display_data_type=Fixed-point  arith_type=Signed (2's comp)  n_bits=16  bin_pt=13  preci_type=Single  exp_width=8  frac_width=24  explicit_period=off  period=1  equ=P=C  opselect=C  inp2=PCIN>>17  opr=+  inp1=P  carry=CIN  dbl_ovrd=off  block_type=constant
  Inverter4 : xbsIndex_r4/Inverter  en=off  latency=0  dbl_ovrd=off  block_type=inv
  Shift6 : xbsIndex_r4/Shift  shift_dir=Right  shift_bits=3  en=off  latency=0  precision=User Defined  arith_type="Signed  (2's comp)"  n_bits=16  bin_pt=13  quantization=Truncate  overflow=Wrap  dbl_ovrd=off  block_type=shift
  Shift7 : xbsIndex_r4/Shift  shift_dir=Right  shift_bits=3  en=off  latency=0  precision=User Defined  arith_type="Signed  (2's comp)"  n_bits=16  bin_pt=13  quantization=Truncate  overflow=Wrap  dbl_ovrd=off  block_type=shift
  Slice5 : xbsIndex_r4/Slice  nbits=1  boolean_output=on  mode=Upper Bit Location + Width  bit1=0  base1=MSB of Input  bit0=0  base0=LSB of Input  dbl_ovrd=off  block_type=slice
  xo : Outport
  yo : Outport  Port=2
  zo : Outport  Port=3
  wires:
  xi/1 -> AddSub10/1, Shift6/1
  yi/1 -> AddSub11/1, Shift7/1
  zi/1 -> AddSub12/1, Slice5/1
  Slice5/1 -> AddSub11/3, Inverter4/1
  Inverter4/1 -> AddSub12/3, AddSub10/3
  AddSub12/1 -> zo/1
  Constant7/1 -> AddSub12/2
  AddSub11/1 -> yo/1
  Shift6/1 -> AddSub11/2
  AddSub10/1 -> xo/1
  Shift7/1 -> AddSub10/2

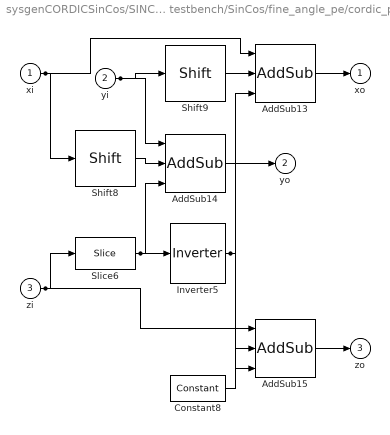
== system sysgenCORDICSinCos/SINCOS testbench/SinCos/fine_angle_pe/cordic_pe4 ==
  xi : Inport
  yi : Inport  Port=2
  zi : Inport  Port=3
  AddSub13 : xbsIndex_r4/AddSub  mode=Addition or Subtraction  use_carryin=off  use_carryout=off  en=off  latency=1  precision=User Defined  arith_type="Signed  (2's comp)"  n_bits=16  bin_pt=13  quantization=Truncate  overflow=Wrap  dbl_ovrd=off  use_behavioral_HDL=off  hw_selection=Fabric  pipelined=off  block_type=addsub
  AddSub14 : xbsIndex_r4/AddSub  mode=Addition or Subtraction  use_carryin=off  use_carryout=off  en=off  latency=1  precision=User Defined  arith_type="Signed  (2's comp)"  n_bits=16  bin_pt=13  quantization=Truncate  overflow=Wrap  dbl_ovrd=off  use_behavioral_HDL=off  hw_selection=Fabric  pipelined=off  block_type=addsub
  AddSub15 : xbsIndex_r4/AddSub  mode=Addition or Subtraction  use_carryin=off  use_carryout=off  en=off  latency=1  precision=User Defined  arith_type="Signed  (2's comp)"  n_bits=16  bin_pt=13  quantization=Truncate  overflow=Wrap  dbl_ovrd=off  use_behavioral_HDL=off  hw_selection=Fabric  pipelined=off  block_type=addsub
  Constant8 : xbsIndex_r4/Constant  const=0.0624188099959574  gui_display_data_type=Fixed-point  arith_type=Signed (2's comp)  n_bits=16  bin_pt=13  preci_type=Single  exp_width=8  frac_width=24  explicit_period=off  period=1  equ=P=C  opselect=C  inp2=PCIN>>17  opr=+  inp1=P  carry=CIN  dbl_ovrd=off  block_type=constant
  Inverter5 : xbsIndex_r4/Inverter  en=off  latency=0  dbl_ovrd=off  block_type=inv
  Shift8 : xbsIndex_r4/Shift  shift_dir=Right  shift_bits=4  en=off  latency=0  precision=User Defined  arith_type="Signed  (2's comp)"  n_bits=16  bin_pt=13  quantization=Truncate  overflow=Wrap  dbl_ovrd=off  block_type=shift
  Shift9 : xbsIndex_r4/Shift  shift_dir=Right  shift_bits=4  en=off  latency=0  precision=User Defined  arith_type="Signed  (2's comp)"  n_bits=16  bin_pt=13  quantization=Truncate  overflow=Wrap  dbl_ovrd=off  block_type=shift
  Slice6 : xbsIndex_r4/Slice  nbits=1  boolean_output=on  mode=Upper Bit Location + Width  bit1=0  base1=MSB of Input  bit0=0  base0=LSB of Input  dbl_ovrd=off  block_type=slice
  xo : Outport
  yo : Outport  Port=2
  zo : Outport  Port=3
  wires:
  xi/1 -> AddSub13/1, Shift8/1
  yi/1 -> AddSub14/1, Shift9/1
  zi/1 -> AddSub15/1, Slice6/1
  Slice6/1 -> AddSub14/3, Inverter5/1
  Inverter5/1 -> AddSub15/3, AddSub13/3
  AddSub15/1 -> zo/1
  Constant8/1 -> AddSub15/2
  AddSub14/1 -> yo/1
  Shift8/1 -> AddSub14/2
  AddSub13/1 -> xo/1
  Shift9/1 -> AddSub13/2

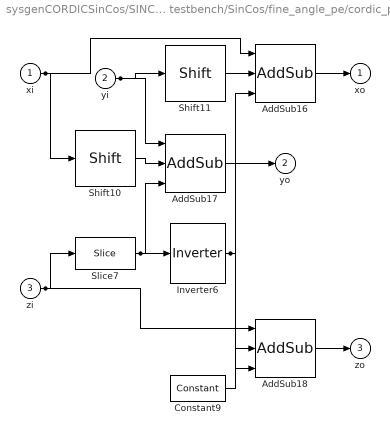
== system sysgenCORDICSinCos/SINCOS testbench/SinCos/fine_angle_pe/cordic_pe5 ==
  xi : Inport
  yi : Inport  Port=2
  zi : Inport  Port=3
  AddSub16 : xbsIndex_r4/AddSub  mode=Addition or Subtraction  use_carryin=off  use_carryout=off  en=off  latency=1  precision=User Defined  arith_type="Signed  (2's comp)"  n_bits=16  bin_pt=13  quantization=Truncate  overflow=Wrap  dbl_ovrd=off  use_behavioral_HDL=off  hw_selection=Fabric  pipelined=off  block_type=addsub
  AddSub17 : xbsIndex_r4/AddSub  mode=Addition or Subtraction  use_carryin=off  use_carryout=off  en=off  latency=1  precision=User Defined  arith_type="Signed  (2's comp)"  n_bits=16  bin_pt=13  quantization=Truncate  overflow=Wrap  dbl_ovrd=off  use_behavioral_HDL=off  hw_selection=Fabric  pipelined=off  block_type=addsub
  AddSub18 : xbsIndex_r4/AddSub  mode=Addition or Subtraction  use_carryin=off  use_carryout=off  en=off  latency=1  precision=User Defined  arith_type="Signed  (2's comp)"  n_bits=16  bin_pt=13  quantization=Truncate  overflow=Wrap  dbl_ovrd=off  use_behavioral_HDL=off  hw_selection=Fabric  pipelined=off  block_type=addsub
  Constant9 : xbsIndex_r4/Constant  const=0.0312398334302683  gui_display_data_type=Fixed-point  arith_type=Signed (2's comp)  n_bits=16  bin_pt=13  preci_type=Single  exp_width=8  frac_width=24  explicit_period=off  period=1  equ=P=C  opselect=C  inp2=PCIN>>17  opr=+  inp1=P  carry=CIN  dbl_ovrd=off  block_type=constant
  Inverter6 : xbsIndex_r4/Inverter  en=off  latency=0  dbl_ovrd=off  block_type=inv
  Shift10 : xbsIndex_r4/Shift  shift_dir=Right  shift_bits=5  en=off  latency=0  precision=User Defined  arith_type="Signed  (2's comp)"  n_bits=16  bin_pt=13  quantization=Truncate  overflow=Wrap  dbl_ovrd=off  block_type=shift
  Shift11 : xbsIndex_r4/Shift  shift_dir=Right  shift_bits=5  en=off  latency=0  precision=User Defined  arith_type="Signed  (2's comp)"  n_bits=16  bin_pt=13  quantization=Truncate  overflow=Wrap  dbl_ovrd=off  block_type=shift
  Slice7 : xbsIndex_r4/Slice  nbits=1  boolean_output=on  mode=Upper Bit Location + Width  bit1=0  base1=MSB of Input  bit0=0  base0=LSB of Input  dbl_ovrd=off  block_type=slice
  xo : Outport
  yo : Outport  Port=2
  zo : Outport  Port=3
  wires:
  xi/1 -> AddSub16/1, Shift10/1
  yi/1 -> AddSub17/1, Shift11/1
  zi/1 -> AddSub18/1, Slice7/1
  Slice7/1 -> AddSub17/3, Inverter6/1
  Inverter6/1 -> AddSub18/3, AddSub16/3
  AddSub18/1 -> zo/1
  Constant9/1 -> AddSub18/2
  AddSub17/1 -> yo/1
  Shift10/1 -> AddSub17/2
  AddSub16/1 -> xo/1
  Shift11/1 -> AddSub16/2

== system sysgenCORDICSinCos/SINCOS testbench/SinCos/fine_angle_pe/cordic_pe6 ==
  xi : Inport
  yi : Inport  Port=2
  zi : Inport  Port=3
  AddSub19 : xbsIndex_r4/AddSub  mode=Addition or Subtraction  use_carryin=off  use_carryout=off  en=off  latency=1  precision=User Defined  arith_type="Signed  (2's comp)"  n_bits=16  bin_pt=13  quantization=Truncate  overflow=Wrap  dbl_ovrd=off  use_behavioral_HDL=off  hw_selection=Fabric  pipelined=off  block_type=addsub
  AddSub20 : xbsIndex_r4/AddSub  mode=Addition or Subtraction  use_carryin=off  use_carryout=off  en=off  latency=1  precision=User Defined  arith_type="Signed  (2's comp)"  n_bits=16  bin_pt=13  quantization=Truncate  overflow=Wrap  dbl_ovrd=off  use_behavioral_HDL=off  hw_selection=Fabric  pipelined=off  block_type=addsub
  AddSub21 : xbsIndex_r4/AddSub  mode=Addition or Subtraction  use_carryin=off  use_carryout=off  en=off  latency=1  precision=User Defined  arith_type="Signed  (2's comp)"  n_bits=16  bin_pt=13  quantization=Truncate  overflow=Wrap  dbl_ovrd=off  use_behavioral_HDL=off  hw_selection=Fabric  pipelined=off  block_type=addsub
  Constant10 : xbsIndex_r4/Constant  const=0.0156237286204768  gui_display_data_type=Fixed-point  arith_type=Signed (2's comp)  n_bits=16  bin_pt=13  preci_type=Single  exp_width=8  frac_width=24  explicit_period=off  period=1  equ=P=C  opselect=C  inp2=PCIN>>17  opr=+  inp1=P  carry=CIN  dbl_ovrd=off  block_type=constant
  Inverter7 : xbsIndex_r4/Inverter  en=off  latency=0  dbl_ovrd=off  block_type=inv
  Shift12 : xbsIndex_r4/Shift  shift_dir=Right  shift_bits=6  en=off  latency=0  precision=User Defined  arith_type="Signed  (2's comp)"  n_bits=16  bin_pt=13  quantization=Truncate  overflow=Wrap  dbl_ovrd=off  block_type=shift
  Shift13 : xbsIndex_r4/Shift  shift_dir=Right  shift_bits=6  en=off  latency=0  precision=User Defined  arith_type="Signed  (2's comp)"  n_bits=16  bin_pt=13  quantization=Truncate  overflow=Wrap  dbl_ovrd=off  block_type=shift
  Slice8 : xbsIndex_r4/Slice  nbits=1  boolean_output=on  mode=Upper Bit Location + Width  bit1=0  base1=MSB of Input  bit0=0  base0=LSB of Input  dbl_ovrd=off  block_type=slice
  xo : Outport
  yo : Outport  Port=2
  zo : Outport  Port=3
  wires:
  xi/1 -> AddSub19/1, Shift12/1
  yi/1 -> AddSub20/1, Shift13/1
  zi/1 -> AddSub21/1, Slice8/1
  Slice8/1 -> AddSub20/3, Inverter7/1
  Inverter7/1 -> AddSub21/3, AddSub19/3
  AddSub21/1 -> zo/1
  Constant10/1 -> AddSub21/2
  AddSub20/1 -> yo/1
  Shift12/1 -> AddSub20/2
  AddSub19/1 -> xo/1
  Shift13/1 -> AddSub19/2
